simulink model "FSK"  (Simulink 8.2)
settings: Solver=ode45  StartTime=0.0  StopTime=10.0  RelTol=1e-3
libraries: dsparch4 x4, commchan3 x1, commrandsrc2 x1, commsink2 x1, dspsigops x1
settings Model: Creator=Yi_Liu  LastModifiedBy=Administrator
settings DataIOCC: SignalLoggingSaveFormat=Dataset
settings OptimizationCC: ExpressionDepthLimit=128
settings DebuggingCC: FcnCallInpInsideContextMsg=EnableAllAsError  StateNameClashWarn=none
settings GRTTargetCC: CombineOutputUpdateFcns=on  GRTInterface=off

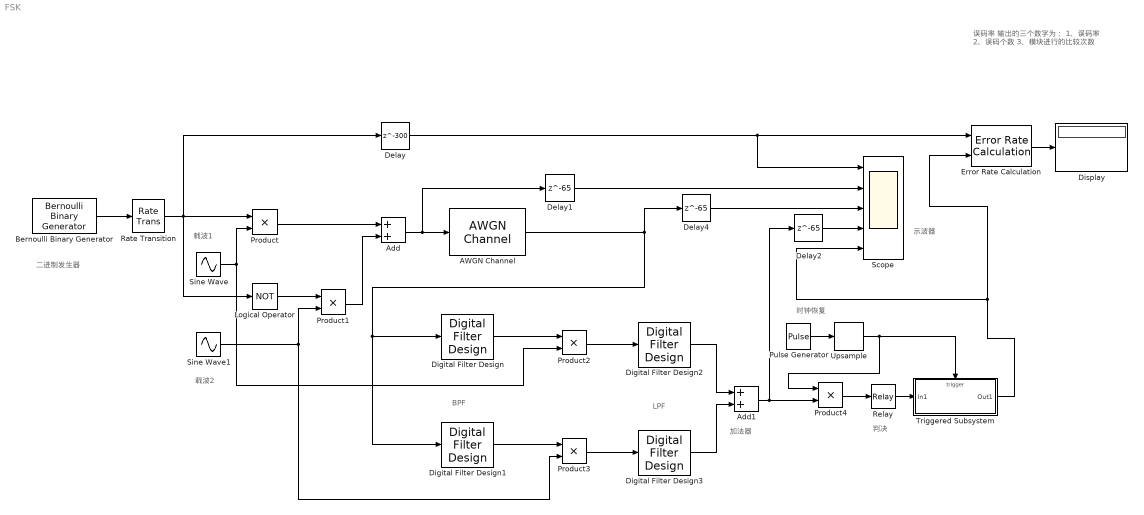
== system FSK ==
  note: 误码率
      | 输出的三个数字为：
      | 1、误码率
      | 2、误码个数
      | 3、模块进行的比较次数
  note: 示波器
  note: LPF
  note: BPF
  note: 加法器
  note: 判决
  note: 时钟恢复
  note: 载波2
  note: 载波1
  note: 二进制发生器
  AWGN Channel : commchan3/AWGN Channel  InputProcessing=Columns as channels (frame based)  seed=67  noiseMode=Variance from mask  EbNodB=10  EsNodB=10  SNRdB=10  bitsPerSym=1  Ps=1  Tsym=1  variance=0.005
  Add : Sum  SampleTime=1/10000
  Add1 : Sum  SampleTime=0.0001
  Bernoulli Binary Generator : commrandsrc2/Bernoulli Binary Generator  P=0.5  seed=61  Ts=1/500  frameBased=off  sampPerFrame=1  orient=off  outDataType=double
  Delay : Delay  DelayLength=300  InitialCondition=0  SampleTime=0.00001
  Delay1 : Delay  DelayLength=65  InitialCondition=0  SampleTime=0.00001
  Delay2 : Delay  DelayLength=65  InitialCondition=0  SampleTime=0.00001
  Delay4 : Delay  DelayLength=65  InitialCondition=0  SampleTime=0.00001
  Digital Filter Design{,1..3} (4 alike) : dsparch4/Digital Filter Design  mwdsp_browser_bugfix_var=off
  Display : Display
  Error Rate Calculation : commsink2/Error Rate Calculation  N=0  st_delay=0  cp_mode=Entire frame  subframe=[]  PMode=Port  WsName=ErrorVec  RsMode2=off  stop=off  numErr=100  maxBits=1e6
  Logical Operator : Logic  Operator=NOT  AllPortsSameDT=off  OutDataTypeStr=boolean
  Product{,1..4} (5 alike) : Product  SampleTime=0.0001
  Pulse Generator : DiscretePulseGenerator  Period=10  PulseWidth=5  SampleTime=1/10000
  Rate Transition : RateTransition  OutPortSampleTime=1/10000
  Relay : Relay  OnSwitchValue=0  OffSwitchValue=0  SampleTime=0.0001
  Scope : Scope  NumInputPorts=5
      settings: YMin=-5~-2~-5~-5~-5  YMax=5~2~5~5~5
  Sine Wave : Sin  Frequency=2*pi*500  SampleTime=1/10000
  Sine Wave1 : Sin  Frequency=2*pi*1000  SampleTime=1/10000
  Triggered Subsystem : Subsystem  TreatAsAtomicUnit=on
  Upsample : dspsigops/Upsample  N=10  phase=0  RateOptions=Allow multirate processing  ic=0  mode=Unused parameter value
  wires:
  Bernoulli Binary Generator/1 -> Rate Transition/1
  Error Rate Calculation/1 -> Display/1
  Sine Wave/1 -> Product/2, Product2/2
  Logical Operator/1 -> Product1/1
  Sine Wave1/1 -> Product3/2, Product1/2
  Product1/1 -> Add/2
  Product/1 -> Add/1
  Add/1 -> Delay1/1, AWGN Channel/1
  AWGN Channel/1 -> Delay4/1, Digital Filter Design1/1, Digital Filter Design/1
  Digital Filter Design/1 -> Product2/1
  Digital Filter Design1/1 -> Product3/1
  Product2/1 -> Digital Filter Design2/1
  Product3/1 -> Digital Filter Design3/1
  Digital Filter Design2/1 -> Add1/1
  Digital Filter Design3/1 -> Add1/2
  Add1/1 -> Delay2/1, Product4/2
  Upsample/1 -> Product4/1, Triggered Subsystem/Trigger
  Pulse Generator/1 -> Upsample/1
  Product4/1 -> Relay/1
  Relay/1 -> Triggered Subsystem/1(In1)
  Triggered Subsystem/1(Out1) -> Scope/5, Error Rate Calculation/2
  Delay1/1 -> Scope/2
  Delay4/1 -> Scope/3
  Delay2/1 -> Scope/4
  Rate Transition/1 -> Delay/1, Product/1, Logical Operator/1
  Delay/1 -> Scope/1, Error Rate Calculation/1

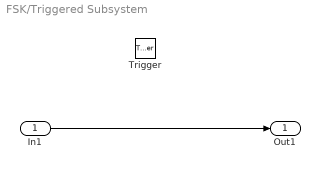
== system FSK/Triggered Subsystem ==
  In1 : Inport
  Trigger : TriggerPort
  Out1 : Outport
  wires:
  In1/1 -> Out1/1
